simulink model "Copy_3_of_InctanceConfig"  (R2023a)
settings: Solver=VariableStepAuto  StartTime=0.0  StopTime=10.0  RelTol=1e-3
undefined symbols (not defined in the file or in its folder): gray
libraries: sim3dautolib x2, sim3dcameralib x1, sim3dlib x1
settings Model: SnapshotInterval=1  Creator=Franz  LastModifiedBy=Franz

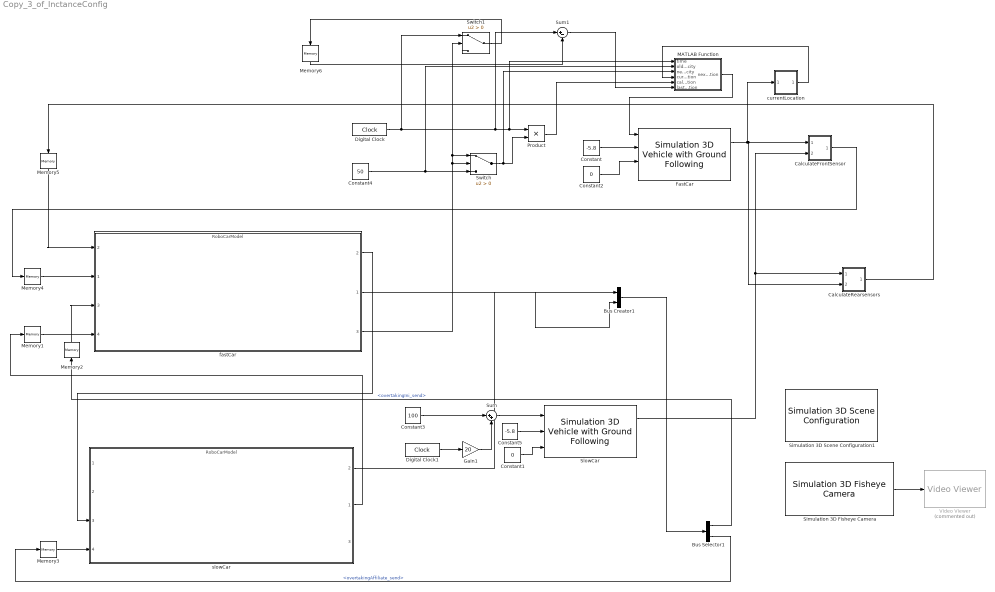
== system Copy_3_of_InctanceConfig ==
  Bus Creator1 : BusCreator  Inputs=2
  Bus Selector1 : BusSelector  OutputSignals=overtakingIni_send,overtakingAffiliate_send
  CalculateFrontSensor : Subsystem
  CalculateRearsensors : Subsystem
  Constant : Constant  Value=-5.8
  Constant1 : Constant  Value=0
  Constant2 : Constant  Value=0
  Constant3 : Constant  Value=100
  Constant4 : Constant  Value=50
  Constant5 : Constant  Value=-5.8
  Digital Clock : DigitalClock  SampleTime=0.01
  Digital Clock1 : DigitalClock  SampleTime=0.01
  FastCar : sim3dautolib/Simulation 3D Vehicle with Ground Following  Priority=-1  PassVehMesh=Muscle car  MeshPath=/MathWorksAutomotiveContent/Vehicles/Muscle/Meshes/SK_MuscleCar.SK_MuscleCar  TrackWidth=1.9  WheelBase=3  WheelRadius=0.35  VehColor=Red  InitialPos=[0,0,0]  InitialRot=[0, 0, 0]  ActorName=FastCar  SampleTime=-1  ActorType=SimulinkVehicle  ID=C  aMode=3  ActorTag=FastCar  CoordinateScheme=ISO  VehLightsControl=on  HeadlightColor=[ 1, 1, 1 ]  HighBeamIntensity=100000  LowBeamIntensity=60000  HighBeamConeAngle=70  LowBeamConeAngle=70  LeftHeadlightOrientation=[ 0, 0 ]  RightHeadlightOrientation=[ 0, 0 ]  BrakelightIntensity=500  ReverselightIntensity=500  SignallightIntensity=500  SignallightPeriod=1  SignalPulseWidth=50  TransformOutportEnabled=on
      settings: LibrarySourceBlock=drivingsim3d/Simulation 3D Vehicle with Ground Following
  Gain1 : Gain  Gain=20
  MATLAB Function : MATLAB Function  TreatAsAtomicUnit=on
  Memory{1..6} (6 alike) : Memory
  Product : Product
  Simulation 3D Fisheye Camera : sim3dcameralib/Simulation 3D Fisheye Camera  Priority=1  sensorTag=Sim3dSensor1  sensorId=1  sensorName=Sim3dSensor1  vehTagList={'FastCar';'Scene Origin';'SlowCar'}  vehTag=FastCar  mountLoc=Roof center  offsetFlag=off  tmountOffset=[0, 0, 0]  extTmount=off  rmountOffset=[0, 0, 0]  extRmount=off  OpticalCenter=[640, 360]  ImageSize=[720, 1280]  RadialDistortion=[320, 0, 0, 0]  StretchMatrix=[1, 0; 0, 1]  TransformOutportEnabled=off  SampleTime=-1  mountPoint=[-0.25 0 1.57000005245209]  mountOrientation=[0 0 0]  aMode=3  ID=1
      settings: LibrarySourceBlock=drivingsim3d/Simulation 3D Fisheye Camera
  Simulation 3D Scene Configuration1 : sim3dlib/Simulation 3D Scene Configuration  Priority=0  ProjectFormat=Default Scenes  SceneDesc=Straight road  ProjectName=D:\Program Files\MATLAB\R2023a\toolbox\shared\sim3d_projects\automotive_project\UE4\WindowsNoEditor\VehicleSimulation.exe  ScenePath=/Game/Maps/HwStrght  EnableOpenDRIVE=off  vehTagList={'FastCar';'Scene Origin';'SlowCar'}  vehTag=FastCar  OpVisEn=off  Ts=1/60  EnableWindow=on  EnableRemoteAccess=off  EnableWeather=off  SunAltitude=40.0  SunAzimuth=90  clouds=10  wind=1  fog=0  rain=0  EnableGeospatial=off  OriginHeight=200  OriginLatitude=40.744652  OriginLongitude=-73.988864  MapStyle=Aerial  AdditionalAssetIDs=[]  UseAdvancedSunSky=off  SolarTime=11  TimeZone=-5  Day=21  Month=9  Year=2022  UseDaylightSavingTime=on  DSTStartDay=10  DSTStartMonth=3  DSTEndDay=3  DSTEndMonth=11  DSTSwitchHour=2  sensorTag=MainCamera2  sensorId=2  sensorName=MainCamera2  mountLoc=Origin  offsetFlag=off  tmountOffset=[0, 0, 0]  rmountOffset=[0, 0, 0]  HorizontalResolution=1280  VerticalResolution=720  HorizontalFOV=60  mountPoint=[0 0 0]  mountOrientation=[0 0 0]  aMode=3  ID=2  GeoTrigger=Inactive
      settings: LibrarySourceBlock=drivingsim3d/Simulation 3D Scene Configuration
  SlowCar : sim3dautolib/Simulation 3D Vehicle with Ground Following  Priority=-1  PassVehMesh=Muscle car  MeshPath=/MathWorksAutomotiveContent/Vehicles/Muscle/Meshes/SK_MuscleCar.SK_MuscleCar  TrackWidth=1.9  WheelBase=3  WheelRadius=0.35  VehColor=Green  InitialPos=[0, 0, 0]  InitialRot=[0, 0, 0]  ActorName=SlowCar  SampleTime=-1  ActorType=SimulinkVehicle  ID=C  aMode=3  ActorTag=SlowCar  CoordinateScheme=ISO  VehLightsControl=off  HeadlightColor=[ 1, 1, 1 ]  HighBeamIntensity=100000  LowBeamIntensity=60000  HighBeamConeAngle=70  LowBeamConeAngle=70  LeftHeadlightOrientation=[ 0, 0 ]  RightHeadlightOrientation=[ 0, 0 ]  BrakelightIntensity=500  ReverselightIntensity=500  SignallightIntensity=500  SignallightPeriod=1  SignalPulseWidth=50  TransformOutportEnabled=on
      settings: LibrarySourceBlock=drivingsim3d/Simulation 3D Vehicle with Ground Following
  Sum : Sum  Inputs=|++
  Sum1 : Sum  Inputs=|+-
  Switch : Switch  Criteria=u2 > Threshold  SaturateOnIntegerOverflow=off  InputSameDT=off
  Switch1 : Switch  Criteria=u2 > Threshold  SaturateOnIntegerOverflow=off  InputSameDT=off
  Video Viewer : VideoViewer  Commented=on  colormapValue=gray(256)  FigPos=[399 900 1271 692]
  currentLocation : Subsystem
  fastCar : ModelReference  ModelNameDialog=RoboCarModel.slx  SimulationMode=Normal  ModelReferenceVersion=1.127
      settings: PortSchema="{\"entries\":[{\"content\":{\"sides\":[{\"content\":{\"connectorIds\":[\"In2\",\"In1\",\"In3\",\"In4\"]},\"type\":\"ConnectorPlacement.EquallySpacedRectSide\",\"uuid\":\"95733cf0-032d-453a-9995-7e8d3e1a24c3\"},{\"content\":{\"connectorIds\":[\"Out2\",\"Out1\",\"Out3\"],\"side\":\"RIGHT\"},\"type\":\"ConnectorPlacement.EquallySpacedRectSide\",\"uuid\":\"8d40af39-e74b-4bad-b693-9b5567a60d93\"},{\"content\":{\"side\":\"TOP\"},\"type\":\"ConnectorPlacement.EquallySpacedRectSide\",\"uuid\":\"43bbd94f-fc32-448c-b6cd-ad2d068142f7\"}]},\"type\":\"ConnectorPlacement.EquallySpacedConnector\",\"uuid\":\"f2b8ce5d-c214-4fd8-985d-570b817192f6\"}],\"packageUris\":[\"http://schema.mathworks.com/mf0/Connector/R2020b\"],\"version\":\"1.0\"}"
  slowCar : ModelReference  ModelNameDialog=RoboCarModel.slx  SimulationMode=Normal  ModelReferenceVersion=1.127
      settings: PortSchema="{\"entries\":[{\"content\":{\"sides\":[{\"content\":{\"connectorIds\":[\"In1\",\"In2\",\"In3\",\"In4\"]},\"type\":\"ConnectorPlacement.EquallySpacedRectSide\",\"uuid\":\"95733cf0-032d-453a-9995-7e8d3e1a24c3\"},{\"content\":{\"connectorIds\":[\"Out2\",\"Out1\",\"Out3\"],\"side\":\"RIGHT\"},\"type\":\"ConnectorPlacement.EquallySpacedRectSide\",\"uuid\":\"8d40af39-e74b-4bad-b693-9b5567a60d93\"},{\"content\":{\"side\":\"TOP\"},\"type\":\"ConnectorPlacement.EquallySpacedRectSide\",\"uuid\":\"43bbd94f-fc32-448c-b6cd-ad2d068142f7\"}]},\"type\":\"ConnectorPlacement.EquallySpacedConnector\",\"uuid\":\"f2b8ce5d-c214-4fd8-985d-570b817192f6\"}],\"packageUris\":[\"http://schema.mathworks.com/mf0/Connector/R2020b\"],\"version\":\"1.0\"}"
  wires:
  Simulation 3D Fisheye Camera/1 -> Video Viewer/1
  fastCar/1 -> Bus Creator1/2
  Constant5/1 -> SlowCar/2
  Constant4/1 -> MATLAB Function/2(oldvelocity), Switch/3
  Constant/1 -> FastCar/2
  Constant2/1 -> FastCar/3
  Constant1/1 -> SlowCar/3
  Constant3/1 -> Sum/1
  Digital Clock1/1 -> Gain1/1
  Gain1/1 -> Sum/2
  Sum/1 -> SlowCar/1
  fastCar/3 -> Switch1/2, Switch/1, Switch/2
  Digital Clock/1 -> Sum1/1, MATLAB Function/1(time), Product/1, Switch1/1
  slowCar/2 -> Bus Creator1/1
  Bus Creator1/1 -> Bus Selector1/1
  Bus Selector1/2 -> Memory3/1  "<overtakingAffiliate_send>"
  Memory1/1 -> fastCar/4
  Memory4/1 -> fastCar/1
  slowCar/1 -> Memory1/1
  Bus Selector1/1 -> Memory2/1  "<overtakingIni_send>"
  fastCar/2 -> slowCar/3
  Memory3/1 -> slowCar/4
  Memory2/1 -> fastCar/3
  FastCar/1 -> CalculateFrontSensor/1(In1), CalculateRearsensors/2(In2), currentLocation/1(In1)
  SlowCar/1 -> CalculateRearsensors/1(In1), CalculateFrontSensor/2(In2)
  CalculateFrontSensor/1(data2) -> Memory4/1
  CalculateRearsensors/1(rearDisctance) -> Memory5/1
  Memory5/1 -> fastCar/2
  Product/1 -> MATLAB Function/5(calculateLocation)
  Switch/1 -> MATLAB Function/3(newVelocity), Product/2
  MATLAB Function/1(nextLocation) -> FastCar/1
  currentLocation/1(data2) -> MATLAB Function/4(currentLocation)
  Switch1/1 -> Memory6/1
  Memory6/1 -> Sum1/2
  Sum1/1 -> MATLAB Function/6(lastlocation)

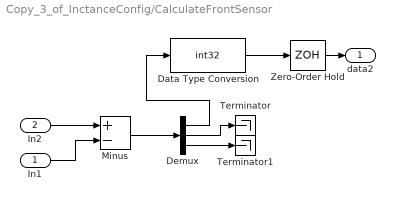
== system Copy_3_of_InctanceConfig/CalculateFrontSensor ==
  In1 : Inport
  In2 : Inport  Port=2
  Data Type Conversion : DataTypeConversion  OutMin=[0]  OutMax=100  OutDataTypeStr=int32  SaturateOnIntegerOverflow=off  RndMeth=Floor
  Demux : Demux  Outputs=3
  Minus : Sum  Inputs=+-  InputSameDT=on  AccumDataTypeStr=int32
  Terminator : Terminator
  Terminator1 : Terminator
  Zero-Order Hold : ZeroOrderHold  SampleTime=0.3
  data2 : Outport
  wires:
  Zero-Order Hold/1 -> data2/1
  Data Type Conversion/1 -> Zero-Order Hold/1
  Demux/2 -> Terminator/1
  Minus/1 -> Demux/1
  Demux/3 -> Terminator1/1
  In1/1 -> Minus/2
  In2/1 -> Minus/1
  Demux/1 -> Data Type Conversion/1

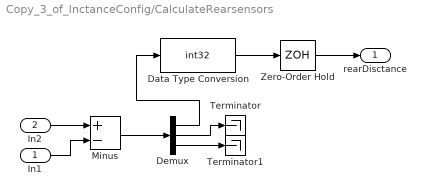
== system Copy_3_of_InctanceConfig/CalculateRearsensors ==
  In1 : Inport
  In2 : Inport  Port=2
  Data Type Conversion : DataTypeConversion  OutMin=[0]  OutMax=100  OutDataTypeStr=int32  SaturateOnIntegerOverflow=off  RndMeth=Floor
  Demux : Demux  Outputs=3
  Minus : Sum  Inputs=+-  InputSameDT=on  AccumDataTypeStr=int32
  Terminator : Terminator
  Terminator1 : Terminator
  Zero-Order Hold : ZeroOrderHold  SampleTime=0.3
  rearDisctance : Outport
  wires:
  Zero-Order Hold/1 -> rearDisctance/1
  Data Type Conversion/1 -> Zero-Order Hold/1
  Demux/2 -> Terminator/1
  Minus/1 -> Demux/1
  Demux/3 -> Terminator1/1
  In1/1 -> Minus/2
  In2/1 -> Minus/1
  Demux/1 -> Data Type Conversion/1

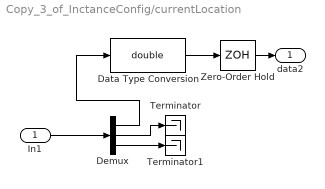
== system Copy_3_of_InctanceConfig/currentLocation ==
  In1 : Inport
  Data Type Conversion : DataTypeConversion  OutMin=[0]  OutMax=100  OutDataTypeStr=double  SaturateOnIntegerOverflow=off  RndMeth=Floor
  Demux : Demux  Outputs=3
  Terminator : Terminator
  Terminator1 : Terminator
  Zero-Order Hold : ZeroOrderHold  SampleTime=0.01
  data2 : Outport
  wires:
  Zero-Order Hold/1 -> data2/1
  Data Type Conversion/1 -> Zero-Order Hold/1
  Demux/2 -> Terminator/1
  Demux/3 -> Terminator1/1
  Demux/1 -> Data Type Conversion/1
  In1/1 -> Demux/1

== matlab function Copy_3_of_InctanceConfig/MATLAB Function ==
  data: time input; nextLocation output; oldvelocity input; newVelocity input; currentLocation input; calculateLocation input; lastlocation input
function nextLocation = fcn(time, oldvelocity, newVelocity, currentLocation, calculateLocation, lastlocation)
    if currentLocation > calculateLocation
        nextLocation = double(lastlocation*oldvelocity + newVelocity*(time - lastlocation));
    else 
        nextLocation = calculateLocation
    end
